simulink model "deadReckoning_heading_start"  (R2017a)
settings: Solver=FixedStepDiscrete  StartTime=0.0  StopTime=10  FixedStep=0.01  RelTol=1e-3
InitFcn:
  | Ts = 0.01;
  | axleLength = 0.28;
  | wheelR = 0.052;
  | ticksPerDeg = 627.2/360;
  | load wheelMotorModel
  | load wheelMotorLUT
undefined symbols (not defined in the file): ticksPerRot
libraries: mobileRoboticsTrainingLib x3
settings Model: Creator=sseshadr  LastModifiedBy=shiremat

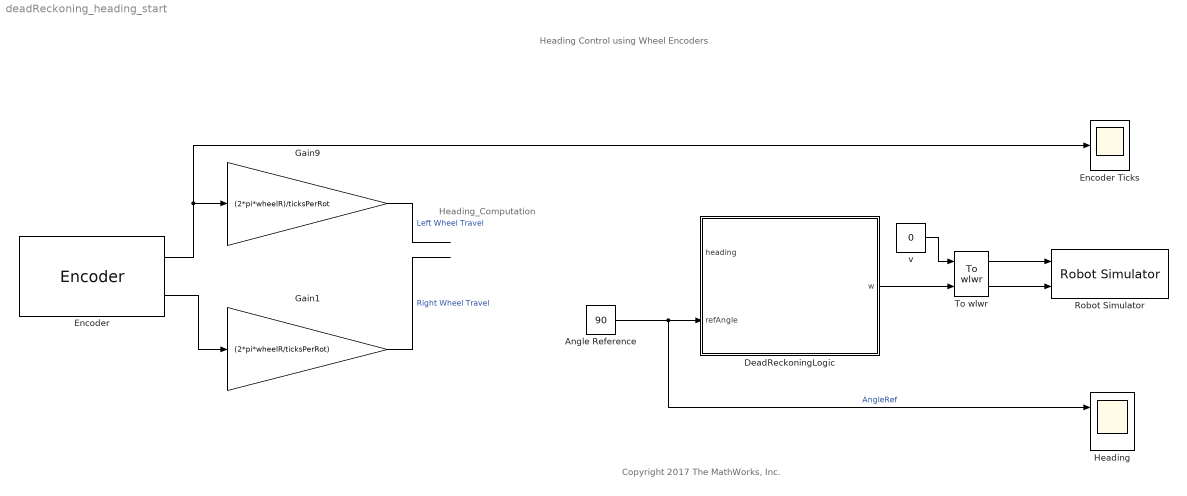
== system deadReckoning_heading_start ==
  note: Heading Control using Wheel Encoders
  note: Heading_Computation
  note: Copyright 2017 The MathWorks, Inc.
  Angle Reference : Constant  Value=90
  DeadReckoningLogic : Stateflow chart  TreatAsAtomicUnit=on
  Encoder : mobileRoboticsTrainingLib/Encoder  axleLength=axleLength  wheelR=wheelR  ticksPerRot=ticksPerRot
      settings: SourceProductName=Mobile Robotics Training Library
  Encoder Ticks : Scope
  Gain1 : Gain  Gain=(2*pi*wheelR/ticksPerRot)
  Gain9 : Gain  Gain=(2*pi*wheelR)/ticksPerRot
  Heading : Scope  NumInputPorts=2
  Robot Simulator : mobileRoboticsTrainingLib/Robot Simulator  Priority=99  mapVar=[]  startX=2  startY=2  startTheta=0  axleLength=axleLength  wheelR=wheelR
  To wlwr : mobileRoboticsTrainingLib/To wlwr  axleLength=0.1  wheelR=0.05
  v : Constant  Value=0
  wires:
  ? -> Heading/2, DeadReckoningLogic/1(heading)  "AngleMeas"
  Gain9/1 -> ?  "Left Wheel Travel"
  Gain1/1 -> ?  "Right Wheel Travel"
  Encoder/1 -> Encoder Ticks/1, Gain9/1
  Encoder/2 -> Gain1/1
  To wlwr/1 -> Robot Simulator/1
  To wlwr/2 -> Robot Simulator/2
  Angle Reference/1 -> Heading/1, DeadReckoningLogic/2(refAngle)  "AngleRef"
  DeadReckoningLogic/1(w) -> To wlwr/2
  v/1 -> To wlwr/1

== stateflow chart deadReckoning_heading_start/DeadReckoningLogic ==
  data: heading input; w output; refAngle input
